simulink model "LQR_Prototype_Tuning"  (R2024a)
settings: Solver=VariableStepAuto  StartTime=0.0  StopTime=80  RelTol=1e-3
values from neighbouring files (symbols this model uses):
  Controller_Continuous = -inv(Input_Matrix_Weight)*Input_Matrix_Ship_Continuous'*Solution_Riccati_Continuous    [LQR_Tuning_Heading_Control.m]
  Ship_Heading_To_Rudder_State_Space_Continuous = ss(State_Matrix_Ship_Continuous,                                                    Input_Matrix_Ship_Continuous,                                                    Measurement_Matrix_Ship_Continuous,                                                    Input_Measurement_Matrix_Ship_Continuous)    [LQR_Tuning_Heading_Control.m]
undefined symbols (not defined in the file or in its folder): DiscIntNeverNeededParam, N_Factor, T_s
settings Model: Creator=gerar  LastModifiedBy=gerar

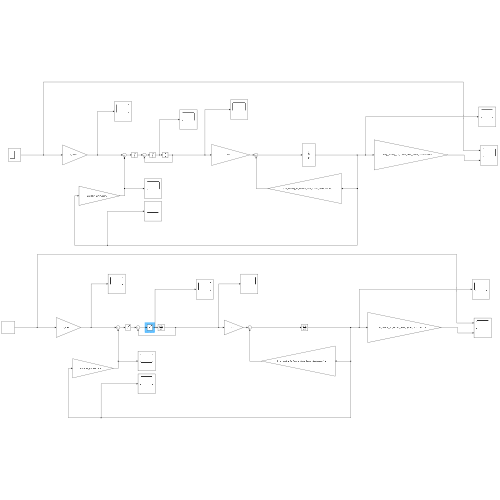
[thumbnail: Simulink's stored preview of the top-level diagram]
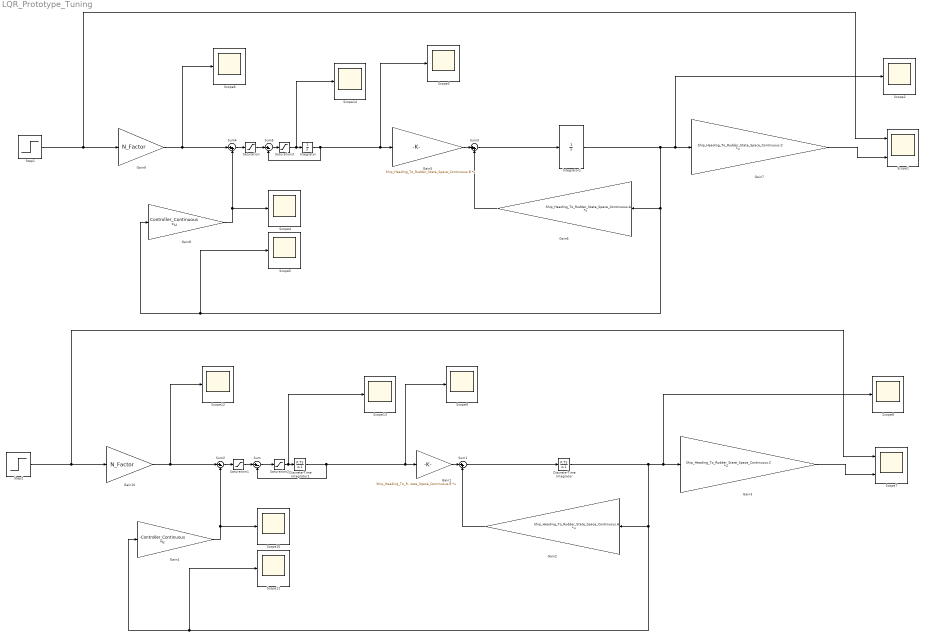
== system LQR_Prototype_Tuning ==
  Discrete-Time Integrator : DiscreteIntegrator  InitialCondition=[0;0]  SampleTime=T_s  ICPrevOutput=DiscIntNeverNeededParam  ICPrevScaledInput=DiscIntNeverNeededParam
  Discrete-Time Integrator1 : DiscreteIntegrator  SampleTime=T_s  ICPrevOutput=DiscIntNeverNeededParam  ICPrevScaledInput=DiscIntNeverNeededParam
  Gain1 : Gain  Gain=Ship_Heading_To_Rudder_State_Space_Continuous.B  Multiplication=Matrix(K*u)
  Gain10 : Gain  Gain=N_Factor
  Gain2 : Gain  Gain=Ship_Heading_To_Rudder_State_Space_Continuous.A  Multiplication=Matrix(K*u)
  Gain3 : Gain  Gain=Ship_Heading_To_Rudder_State_Space_Continuous.C  Multiplication=Matrix(K*u)
  Gain4 : Gain  Gain=-Controller_Continuous  Multiplication=Matrix(K*u)
  Gain5 : Gain  Gain=Ship_Heading_To_Rudder_State_Space_Continuous.B  Multiplication=Matrix(K*u)
  Gain6 : Gain  Gain=Ship_Heading_To_Rudder_State_Space_Continuous.A  Multiplication=Matrix(K*u)
  Gain7 : Gain  Gain=Ship_Heading_To_Rudder_State_Space_Continuous.C  Multiplication=Matrix(K*u)
  Gain8 : Gain  Gain=Controller_Continuous  Multiplication=Matrix(K*u)
  Gain9 : Gain  Gain=N_Factor
  Integrator : Integrator
  Integrator1 : Integrator  InitialCondition=[0;0]
  Saturation : Saturate  UpperLimit=+35*(pi/180)  LowerLimit=-35*(pi/180)
  Saturation1 : Saturate  UpperLimit=+35*(pi/180)  LowerLimit=-35*(pi/180)
  Saturation2 : Saturate  UpperLimit=1*(pi/180)  LowerLimit=-1*(pi/180)
  Saturation3 : Saturate  UpperLimit=7*(pi/180)  LowerLimit=-7*(pi/180)
  Scope1 : Scope  NumInputPorts=2
  Scope{2..6,8..14} (12 alike) : Scope
  Scope7 : Scope  NumInputPorts=2
  Step1 : Step  After=50*(pi/180)  SampleTime=0
  Step2 : Step  After=50*(pi/180)  SampleTime=0
  Sum : Sum  Inputs=|+-
  Sum1 : Sum  Inputs=|++
  Sum2 : Sum  Inputs=|+-
  Sum3 : Sum  Inputs=|++
  Sum4 : Sum  Inputs=|++
  Sum5 : Sum  Inputs=|+-
  wires:
  Sum4/1 -> Saturation/1
  Gain9/1 -> Scope6/1, Sum4/1
  Gain7/1 -> Scope1/2
  Gain6/1 -> Sum3/2
  Sum3/1 -> Integrator1/1
  Integrator1/1 -> Gain6/1, Scope5/1, Gain8/1, Scope2/1, Gain7/1
  Gain5/1 -> Sum3/1
  Gain8/1 -> Scope4/1, Sum4/2
  Step1/1 -> Scope1/1, Gain9/1
  Gain2/1 -> Sum1/2
  Sum2/1 -> Saturation1/1
  Gain3/1 -> Scope7/2
  Discrete-Time Integrator/1 -> Gain2/1, Scope11/1, Gain4/1, Scope8/1, Gain3/1
  Gain10/1 -> Scope12/1, Sum2/1
  Gain1/1 -> Sum1/1
  Step2/1 -> Scope7/1, Gain10/1
  Sum1/1 -> Discrete-Time Integrator/1
  Gain4/1 -> Scope10/1, Sum2/2
  Saturation2/1 -> Scope13/1, Discrete-Time Integrator1/1
  Sum/1 -> Saturation2/1
  Saturation1/1 -> Sum/1
  Discrete-Time Integrator1/1 -> Sum/2, Scope9/1, Gain1/1
  Saturation3/1 -> Scope14/1, Integrator/1
  Integrator/1 -> Scope3/1, Gain5/1, Sum5/2
  Sum5/1 -> Saturation3/1
  Saturation/1 -> Sum5/1
